simulink library "lib_dsphdlutils_v2"  (R2019b)
settings: Solver=ode45  StartTime=0.0  StopTime=10.0  RelTol=1e-3  EnableMultiTasking=on
libraries: simulink x8, dspstat3 x5, dspmathops x5
settings Model: Creator=mbabst  LastModifiedBy=mbabst
settings DataIOCC: LimitDataPoints=on
settings OptimizationCC: LifeSpan=inf
settings DebuggingCC: AllowSymbolicDim=off  SFUnexpectedBacktrackingDiag=warning  SFNoUnconditionalDefaultTransitionDiag=warning  SFExecutionAtInitializationDiag=none  ArithmeticOperatorsInVariantConditions=warning
settings SFSimCC: SimUseLocalCustomCode=off  CustomCodeUndefinedFunction=UseInterfaceOnly
settings RTWCC: RTWUseLocalCustomCode=off
settings CodeAppCC: StateflowObjectComments=on
settings GRTTargetCC: TargetLangStandard=C89/C90 (ANSI)  GeneratePreprocessorConditionals=Disable all
settings ConfigComp: CovMetricSettings=dw  CovHtmlReporting=on  CovSaveCumulativeToWorkspaceVar=on  CovSaveSingleToWorkspaceVar=on  CovExternalEMLEnable=off

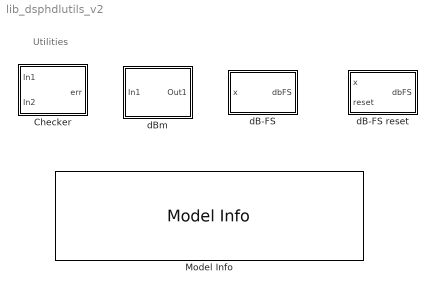
== system lib_dsphdlutils_v2 ==
  note: Utilities
  Checker : Subsystem  mask(Compare two signals){StopSim=on}
      mask prompts: StopSim "Stop Sim on Error"
      mask help:
      | Compare two signals and output the error.
      | If selected, the simulation can be stopped if there is a mismatch.
      mask init:
      | set_param([gcb '/Assertion' ], 'StopWhenAssertionFail', StopSim);
      | set_param([gcb '/Assertion' ], 'Enabled', StopSim);
      mask Display:
      | if StopSim
      |     disp('Compare\n(halt)');
      | else
      |     disp('Compare');
      | end
  Model Info : simulink/Model-Wide Utilities/Model Info  Frame=on  DisplayStringWithTags=|  HorizontalTextAlignment=Left  LeftAlignmentValue=0.02
      | Copyright (c) 2005-2021 DSPlogic, Inc.
      | Distributed under the terms of the Simplified BSD License.
      | The full license is in the file LICENSE, distributed with this software.
      | 
      | Model: %<ModelName> (v%<ModelVersion>)
      | Author: Michael Babst <mike.babst@dsplogic.com>
      | Created: by %<Creator> on %<Created>
      | Modified: by %<ModifiedBy> on %<LastModificationDate>
  dB-FS : Subsystem  mask(Signal level (dB-FS)){}
      mask help: This block computes the running average signal level in decibels with respect to full-scale.
      mask init:
      | units = 'dB';
      | rohms = 1;
      | dispstr = ['dB-FS\n'];
      | %set_param([gcb '/dBconvert'], 'dBtype', 'dB');
      settings: PermitHierarchicalResolution=None
      mask Display: disp(dispstr);
  dB-FS reset : Subsystem  mask(Signal level (dB-FS)){}
      mask help: This block computes the running average signal level in decibels with respect to full-scale.
      mask init:
      | units = 'dB';
      | rohms = 1;
      | dispstr = ['dB-FS\n'];
      | %set_param([gcb '/dBconvert'], 'dBtype', 'dB');
      settings: PermitHierarchicalResolution=None
      mask Display: disp(dispstr);
  dBm : Subsystem  mask(Signal level (dB)){units=dB, rohms=1}
      mask prompts: rohms "Reference Load (ohms)"
      mask help: This block computes the running average signal level in decibels.
      mask init:
      | switch units
      |     case 1
      |         dispstr = ['dB\n(' num2str(rohms) ' ohm)'];
      |         set_param([gcb '/dBconvert'], 'dBtype', 'dB');
      |     case 2
      |         dispstr = ['dBm\n(' num2str(rohms) ' ohm)'];
      |         set_param([gcb '/dBconvert'], 'dBtype', 'dBm');
      | end
      settings: PermitHierarchicalResolution=None
      mask TypeOptions units: dB | dBm
      mask Display: disp(dispstr);

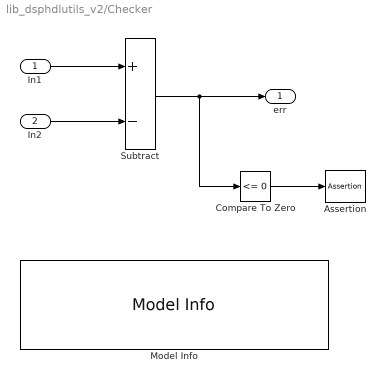
== system lib_dsphdlutils_v2/Checker ==
  In1 : Inport
  In2 : Inport  Port=2
  Assertion : Assertion
      settings: AttributesFormatString=|
      | %<BlockType>
      | %<StopWhenAssertionFail>
  Compare To Zero : simulink/Logic and Bit Operations/Compare To Zero  relop=<=  OutDataTypeStr=boolean
  Model Info : simulink/Model-Wide Utilities/Model Info  Frame=on  DisplayStringWithTags=|  HorizontalTextAlignment=Left  LeftAlignmentValue=0.02
      | Copyright (c) 2005-2021 DSPlogic, Inc.
      | Distributed under the terms of the Simplified BSD License.
      | The full license is in the file LICENSE, distributed with this software.
      | 
      | Model: %<ModelName> (v%<ModelVersion>)
      | Author: Michael Babst <mike.babst@dsplogic.com>
      | Created: by %<Creator> on %<Created>
      | Modified: by %<ModifiedBy> on %<LastModificationDate>
  Subtract : Sum  Inputs=+-
  err : Outport
  wires:
  Compare To Zero/1 -> Assertion/1
  In1/1 -> Subtract/1
  In2/1 -> Subtract/2
  Subtract/1 -> Compare To Zero/1, err/1

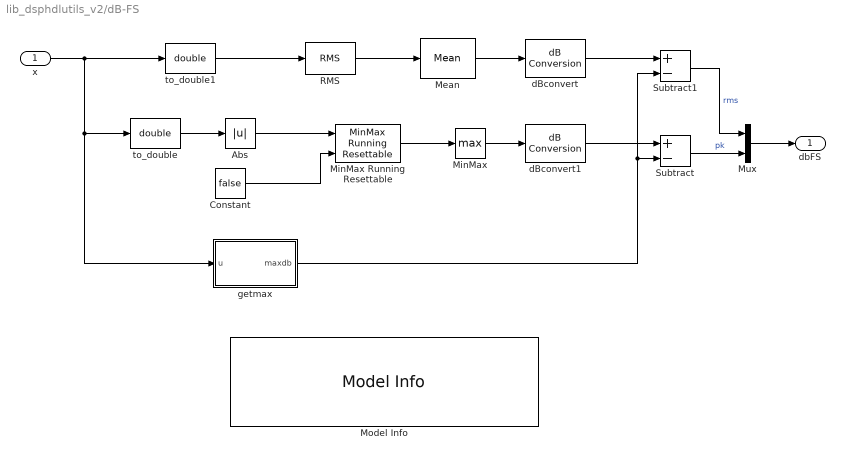
== system lib_dsphdlutils_v2/dB-FS ==
  x : Inport
  Abs : Abs
  Constant : Constant  Value=false  SampleTime=-1
  Mean : dspstat3/Mean  run=off  InputProcessing=Columns as channels (frame based)  reset_popup=None  directionMode=Each column  dimension=1  roiEnable=off  roiType=Rectangles  roiPortion=Entire ROI  roiOutput=Individual statistics for each ROI  roiFlag=off  roundingMode=Floor  overflowMode=off  outputDataTypeStr=Inherit: Same as accumulator  outputMin=[]  outputMax=[]  outputLastDataTypeStr=Inherit: Same as accumulator
  MinMax : MinMax  Function=max
  MinMax Running Resettable : simulink/Math Operations/MinMax Running Resettable  Function=max  vinit=0.0
  Model Info : simulink/Model-Wide Utilities/Model Info  Frame=on  DisplayStringWithTags=|  HorizontalTextAlignment=Left  LeftAlignmentValue=0.02
      | Copyright (c) 2005-2021 DSPlogic, Inc.
      | Distributed under the terms of the Simplified BSD License.
      | The full license is in the file LICENSE, distributed with this software.
      | 
      | Model: %<ModelName> (v%<ModelVersion>)
      | Author: Michael Babst <mike.babst@dsplogic.com>
      | Created: by %<Creator> on %<Created>
      | Modified: by %<ModifiedBy> on %<LastModificationDate>
  Mux : Mux  Inputs=2
  RMS : dspstat3/RMS  run=on  directionMode=Entire input  dimension=1  InputProcessing=Columns as channels (frame based)  reset_popup=None
  Subtract : Sum  Inputs=+-
  Subtract1 : Sum  Inputs=+-
  dBconvert : dspmathops/dB Conversion  dBtype=dB  intype=Amplitude  R=rohms  fuzz=on
      settings: SourceProductName=DSP System Toolbox
  dBconvert1 : dspmathops/dB Conversion  dBtype=dB  intype=Amplitude  R=rohms  fuzz=on
      settings: SourceProductName=DSP System Toolbox
  getmax : MATLAB Function  TreatAsAtomicUnit=on
  to_double : DataTypeConversion  OutDataTypeStr=double
  to_double1 : DataTypeConversion  OutDataTypeStr=double
  dbFS : Outport
  wires:
  Mean/1 -> dBconvert/1
  to_double1/1 -> RMS/1
  to_double/1 -> Abs/1
  Abs/1 -> MinMax Running Resettable/1
  MinMax Running Resettable/1 -> MinMax/1
  getmax/1(maxdb) -> Subtract1/2, Subtract/2
  Constant/1 -> MinMax Running Resettable/2
  x/1 -> getmax/1(u), to_double/1, to_double1/1
  RMS/1 -> Mean/1
  dBconvert/1 -> Subtract1/1
  dBconvert1/1 -> Subtract/1
  Subtract1/1 -> Mux/1  "rms"
  Subtract/1 -> Mux/2  "pk"
  Mux/1 -> dbFS/1
  MinMax/1 -> dBconvert1/1

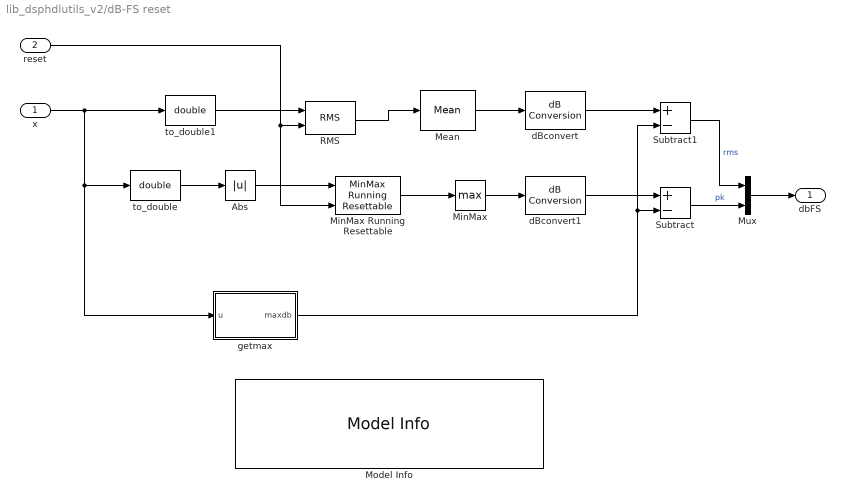
== system lib_dsphdlutils_v2/dB-FS reset ==
  x : Inport
  reset : Inport  Port=2
  Abs : Abs
  Mean : dspstat3/Mean  run=off  InputProcessing=Columns as channels (frame based)  reset_popup=None  directionMode=Each column  dimension=1  roiEnable=off  roiType=Rectangles  roiPortion=Entire ROI  roiOutput=Individual statistics for each ROI  roiFlag=off  roundingMode=Floor  overflowMode=off  outputDataTypeStr=Inherit: Same as accumulator  outputMin=[]  outputMax=[]  outputLastDataTypeStr=Inherit: Same as accumulator
  MinMax : MinMax  Function=max
  MinMax Running Resettable : simulink/Math Operations/MinMax Running Resettable  Function=max  vinit=0.0
  Model Info : simulink/Model-Wide Utilities/Model Info  Frame=on  DisplayStringWithTags=|  HorizontalTextAlignment=Left  LeftAlignmentValue=0.02
      | Copyright (c) 2005-2021 DSPlogic, Inc.
      | Distributed under the terms of the Simplified BSD License.
      | The full license is in the file LICENSE, distributed with this software.
      | 
      | Model: %<ModelName> (v%<ModelVersion>)
      | Author: Michael Babst <mike.babst@dsplogic.com>
      | Created: by %<Creator> on %<Created>
      | Modified: by %<ModifiedBy> on %<LastModificationDate>
  Mux : Mux  Inputs=2
  RMS : dspstat3/RMS  run=on  directionMode=Entire input  dimension=1  InputProcessing=Columns as channels (frame based)  reset_popup=Non-zero sample
  Subtract : Sum  Inputs=+-
  Subtract1 : Sum  Inputs=+-
  dBconvert : dspmathops/dB Conversion  dBtype=dB  intype=Amplitude  R=rohms  fuzz=on
      settings: SourceProductName=DSP System Toolbox
  dBconvert1 : dspmathops/dB Conversion  dBtype=dB  intype=Amplitude  R=rohms  fuzz=on
      settings: SourceProductName=DSP System Toolbox
  getmax : MATLAB Function  TreatAsAtomicUnit=on
  to_double : DataTypeConversion  OutDataTypeStr=double
  to_double1 : DataTypeConversion  OutDataTypeStr=double
  dbFS : Outport
  wires:
  Mean/1 -> dBconvert/1
  to_double1/1 -> RMS/1
  to_double/1 -> Abs/1
  Abs/1 -> MinMax Running Resettable/1
  MinMax Running Resettable/1 -> MinMax/1
  getmax/1(maxdb) -> Subtract1/2, Subtract/2
  reset/1 -> MinMax Running Resettable/2, RMS/2
  x/1 -> getmax/1(u), to_double/1, to_double1/1
  RMS/1 -> Mean/1
  dBconvert/1 -> Subtract1/1
  dBconvert1/1 -> Subtract/1
  Subtract1/1 -> Mux/1  "rms"
  Subtract/1 -> Mux/2  "pk"
  Mux/1 -> dbFS/1
  MinMax/1 -> dBconvert1/1

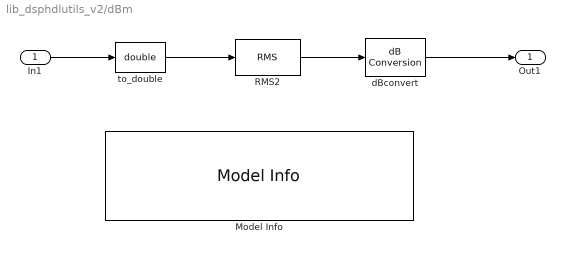
== system lib_dsphdlutils_v2/dBm ==
  In1 : Inport
  Model Info : simulink/Model-Wide Utilities/Model Info  Frame=on  DisplayStringWithTags=|  HorizontalTextAlignment=Left  LeftAlignmentValue=0.02
      | Copyright (c) 2005-2021 DSPlogic, Inc.
      | Distributed under the terms of the Simplified BSD License.
      | The full license is in the file LICENSE, distributed with this software.
      | 
      | Model: %<ModelName> (v%<ModelVersion>)
      | Author: Michael Babst <mike.babst@dsplogic.com>
      | Created: by %<Creator> on %<Created>
      | Modified: by %<ModifiedBy> on %<LastModificationDate>
  RMS2 : dspstat3/RMS  run=on  directionMode=Each column  dimension=1  reset_popup=None
  dBconvert : dspmathops/dB Conversion  dBtype=dB  intype=Amplitude  R=rohms  fuzz=off
      settings: SourceProductName=DSP System Toolbox
  to_double : DataTypeConversion  OutDataTypeStr=double
  Out1 : Outport
  wires:
  In1/1 -> to_double/1
  dBconvert/1 -> Out1/1
  RMS2/1 -> dBconvert/1
  to_double/1 -> RMS2/1

== matlab function lib_dsphdlutils_v2/dB-FS reset/getmax ==
  data: u input; maxdb output
function maxdb  = fcn(u)

persistent proto;
persistent maxmag_dB;

if isempty(proto)
    % Hack so block doesn't bomb when floating point.
    if ~isfloat(u)
        nt_in = numerictype(u);
    else
        nt_in = numerictype(fi(0,0,16,0));
    end        
    proto = fi(0, nt_in);
    hi = upperbound(proto);
    lo = lowerbound(proto); 
    maxmag = double(max(abs(hi),abs(lo)));
    maxmag_dB = 20*log10(maxmag);
end    

maxdb = maxmag_dB;

== matlab function lib_dsphdlutils_v2/dB-FS/getmax ==
  data: u input; maxdb output
function maxdb  = fcn(u)

persistent proto;
persistent maxmag_dB;

if isempty(proto)
    % Hack so block doesn't bomb when floating point.
    if ~isfloat(u)
        nt_in = numerictype(u);
    else
        nt_in = numerictype(fi(0,0,16,0));
    end        
    proto = fi(0, nt_in);
    hi = upperbound(proto);
    lo = lowerbound(proto); 
    maxmag = double(max(abs(hi),abs(lo)));
    maxmag_dB = 20*log10(maxmag);
end    

maxdb = maxmag_dB;
